simulink model "controlled_plant"  (R2018b)
settings: Solver=VariableStepAuto  StartTime=0.0  StopTime=10.0  RelTol=1e-3
settings Model: Creator=Master Broda  LastModifiedBy=Master Broda

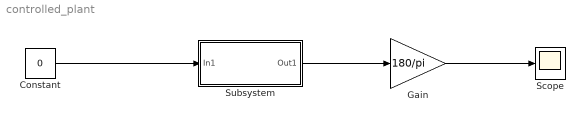
== system controlled_plant ==
  Constant : Constant  Value=0
  Gain : Gain  Gain=180/pi
  Scope : Scope
  Subsystem : Subsystem
  wires:
  Subsystem/1(Out1) -> Gain/1
  Constant/1 -> Subsystem/1(In1)
  Gain/1 -> Scope/1

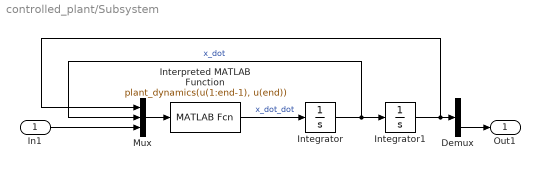
== system controlled_plant/Subsystem ==
  In1 : Inport
  Demux : Demux  Outputs=2
  Integrator : Integrator
  Integrator1 : Integrator
  Interpreted MATLAB Function : MATLABFcn  MATLABFcn=plant_dynamics(u(1:end-1), u(end))  OutputDimensions=2
  Mux : Mux  Inputs=3
  Out1 : Outport
  wires:
  Mux/1 -> Interpreted MATLAB Function/1
  Interpreted MATLAB Function/1 -> Integrator/1  "x_dot_dot"
  In1/1 -> Mux/3
  Integrator/1 -> Mux/2, Integrator1/1  "x_dot"
  Integrator1/1 -> Mux/1, Demux/1
  Demux/2 -> Out1/1
